simulink model "deci_hspice"  (Simulink 7.9)
settings: Solver=ode5  SolverMode=SingleTasking  StartTime=0  StopTime=Tstop  FixedStep=1/fs  RelTol=1e-3  AbsTol=1e-6
values from neighbouring files (symbols this model uses):
  fs4 = fs./OSR    [deci_hspice1_20260927.m]
  G = 2.^-27    (= 7.45058059692e-09)    [deci_hspice1_20260927.m]
  Ts = 1/fs    [build_dsm_decim_model.m]    (also in deci_hspice1_20260927.m = 8.33333333333e-08)
  Ts4 = 1./fs4    [deci_hspice1_20260927.m]
settings Model: Creator=don  LastModifiedBy=Joey.Cheng  ExtModeTrigMode=oneshot  ExtModeArmWhenConnect=off
settings DataIOCC: LimitDataPoints=off  SaveOutput=off  SaveTime=off
settings OptimizationCC: BlockReduction=off  BooleanDataType=off  RollThreshold=2
settings DebuggingCC: SaveWithParameterizedLinksMsg=none  SignalResolutionControl=TryResolveAllWithWarning  SolverPrmCheckMsg=none  MultiTaskDSMMsg=warning  MultiTaskCondExecSysMsg=none  IntegerOverflowMsg=none  FcnCallInpInsideContextMsg=Use local settings  StrictBusMsg=None
settings HardwareCC: TargetUnknown=on
settings RTWCC: IncludeERTFirstTime=on
settings GRTTargetCC: CombineOutputUpdateFcns=off  GRTInterface=on
settings SimEventsCC: propDiagAttribOutput=1  propDiagFcnCallOutput=1  propDiagStatOutput=0  propPreventDuplicateEvents=0

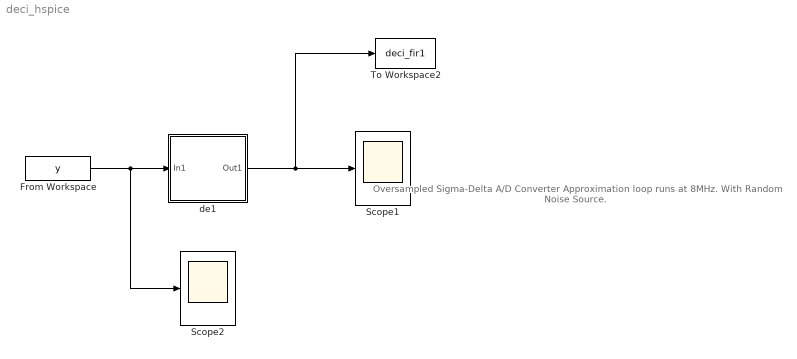
== system deci_hspice ==
  note: Oversampled Sigma-Delta A/D Converter
      | Approximation loop runs at 8MHz.
      | With Random Noise Source.
  From Workspace : FromWorkspace  VariableName=y  OutDataTypeStr=double  SampleTime=Ts
  Scope1 : Scope
      settings: YMin=0  YMax=1
  Scope2 : Scope
      settings: YMin=0  YMax=1
  To Workspace2 : ToWorkspace  VariableName=deci_fir1  SampleTime=1/fs4
  de1 : Subsystem
  wires:
  From Workspace/1 -> Scope2/1, de1/1(In1)
  de1/1(Out1) -> To Workspace2/1, Scope1/1

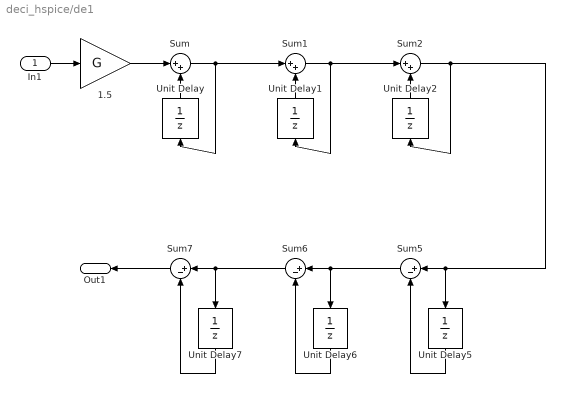
== system deci_hspice/de1 ==
  In1 : Inport  SampleTime=Ts
  1.5 : Gain  Gain=G  SampleTime=Ts  OutDataTypeStr=Inherit: Same as input  ParamDataTypeStr=Inherit: Same as input
  Sum : Sum  Inputs=|++  SaturateOnIntegerOverflow=on  InputSameDT=on  OutDataTypeStr=Inherit: Same as first input
  Sum1 : Sum  Inputs=|++  SaturateOnIntegerOverflow=on  InputSameDT=on  OutDataTypeStr=Inherit: Same as first input
  Sum2 : Sum  Inputs=|++  SaturateOnIntegerOverflow=on  InputSameDT=on  OutDataTypeStr=Inherit: Same as first input
  Sum5 : Sum  Inputs=|+-  SaturateOnIntegerOverflow=on  InputSameDT=on  OutDataTypeStr=Inherit: Same as first input
  Sum6 : Sum  Inputs=|+-  SaturateOnIntegerOverflow=on  InputSameDT=on  OutDataTypeStr=Inherit: Same as first input
  Sum7 : Sum  Inputs=|+-  SaturateOnIntegerOverflow=on  InputSameDT=on  OutDataTypeStr=Inherit: Same as first input
  Unit Delay : UnitDelay  SampleTime=Ts
  Unit Delay1 : UnitDelay  SampleTime=Ts
  Unit Delay2 : UnitDelay  SampleTime=Ts
  Unit Delay5 : UnitDelay  SampleTime=Ts4
  Unit Delay6 : UnitDelay  SampleTime=Ts4
  Unit Delay7 : UnitDelay  SampleTime=Ts4
  Out1 : Outport  SampleTime=1/fs4
  wires:
  Unit Delay/1 -> Sum/2
  Sum/1 -> Sum1/1, Unit Delay/1
  Unit Delay1/1 -> Sum1/2
  Sum1/1 -> Sum2/1, Unit Delay1/1
  Sum2/1 -> Unit Delay2/1, Sum5/1, Unit Delay5/1
  Unit Delay2/1 -> Sum2/2
  Sum5/1 -> Sum6/1, Unit Delay6/1
  Sum6/1 -> Sum7/1, Unit Delay7/1
  Sum7/1 -> Out1/1
  Unit Delay7/1 -> Sum7/2
  Unit Delay6/1 -> Sum6/2
  Unit Delay5/1 -> Sum5/2
  In1/1 -> 1.5/1
  1.5/1 -> Sum/1
